simulink model "realtime_monitor"  (R2025b)
settings: Solver=FixedStepDiscrete  StartTime=0.0  StopTime=10.0  FixedStep=1/360  RelTol=1e-3
undefined symbols (not defined in the file): a, b, b_integ, DiscIntNeverNeededParam
libraries: simulink x3
settings Model: Creator=Hüma  LastModifiedBy=Hüma

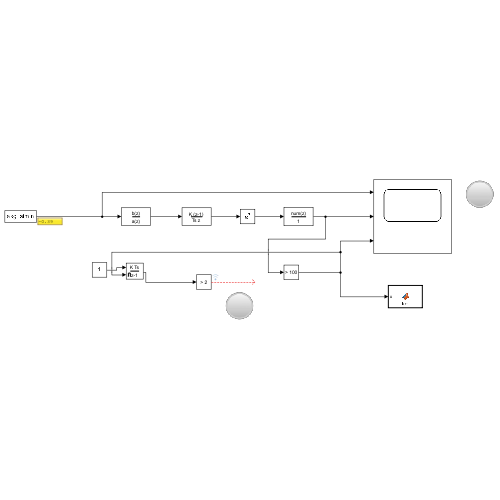
[thumbnail: Simulink's stored preview of the top-level diagram]
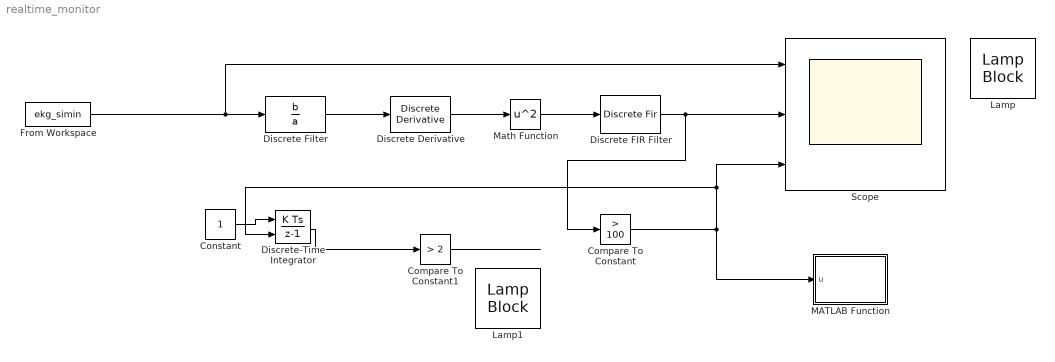
== system realtime_monitor ==
  Compare To Constant : simulink/Logic and Bit Operations/Compare To Constant  relop=>  const=100  OutDataTypeStr=boolean
  Compare To Constant1 : simulink/Logic and Bit Operations/Compare To Constant  relop=>  const=2  OutDataTypeStr=boolean
  Constant : Constant
  Discrete Derivative : simulink/Discrete/Discrete Derivative  gainval=1.0  ICPrevScaledInput=0.0  OutMin=[]  OutMax=[]  OutDataType=fixdt(1, 16)  OutScaling=2^-10  DoSatur=off
  Discrete FIR Filter : DiscreteFir  Coefficients=b_integ
  Discrete Filter : DiscreteFilter  Numerator=b  Denominator=a
  Discrete-Time Integrator : DiscreteIntegrator  ExternalReset=level  SampleTime=-1  ICPrevOutput=DiscIntNeverNeededParam  ICPrevScaledInput=DiscIntNeverNeededParam
  From Workspace : FromWorkspace  VariableName=ekg_simin  OutputAfterFinalValue=Setting to zero
  Lamp : LampBlock  LabelPosition=Hide  DefaultColor=[192.0, 192.0, 192.0]
  Lamp1 : LampBlock  LabelPosition=Hide  DefaultColor=[162.0, 20.0, 47.0]
  MATLAB Function : MATLAB Function  TreatAsAtomicUnit=on
  Math Function : Math  Operator=square
  Scope : Scope  NumInputPorts=3
      settings: ActiveDisplayYMinimum=-48.019454861772388  ActiveDisplayYMaximum=432.17525329494811
  wires:
  From Workspace/1 -> Discrete Filter/1, Scope/1
  Discrete Filter/1 -> Discrete Derivative/1
  Discrete Derivative/1 -> Math Function/1
  Math Function/1 -> Discrete FIR Filter/1
  Discrete FIR Filter/1 -> Scope/2, Compare To Constant/1
  Compare To Constant/1 -> Scope/3, Discrete-Time Integrator/2, MATLAB Function/1(u)
  Constant/1 -> Discrete-Time Integrator/1
  Discrete-Time Integrator/1 -> Compare To Constant1/1
  Compare To Constant1/1 -> ?

== matlab function realtime_monitor/MATLAB Function ==
  data: u input
function fcn(u)
    % Define 'sound' as an extrinsic function to access audio hardware
    coder.extrinsic('sound');
    
    % Persistent variables to store state between simulation steps
    persistent counter;
    persistent last_beep_time;
    
    % Initialize variables at the start of simulation
    if isempty(counter)
        counter = 0;
        last_beep_time = -500; % Ensure system is ready to beep immediately
    end
    
    % Increment counter at every simulation step
    counter = counter + 1;
    
    % LOGIC: 
    % 1. Is the signal High (Pulse detected)?
    % 2. Has enough time passed since the last beep? (Debouncing to prevent audio lock)
    if (double(u) > 0.5) && ((counter - last_beep_time) > 100)
        
        % Generate a clean 1000Hz "Beep" tone
        Fs = 8192;              % Sample rate
        t = 0:1/Fs:0.15;        % Duration: 0.15 seconds
        beep_tone = 0.5 * sin(2*pi*1000*t); 
        
        % Play the sound
        sound(beep_tone, Fs);
        
        % Update the timestamp of the last beep
        last_beep_time = counter;
    end
end
